simulink model "DOB_practice"  (R2021a)
settings: Solver=VariableStepAuto  StartTime=0.0  StopTime=20  RelTol=1e-3
settings Model: Creator=pyi12  LastModifiedBy=pyi12

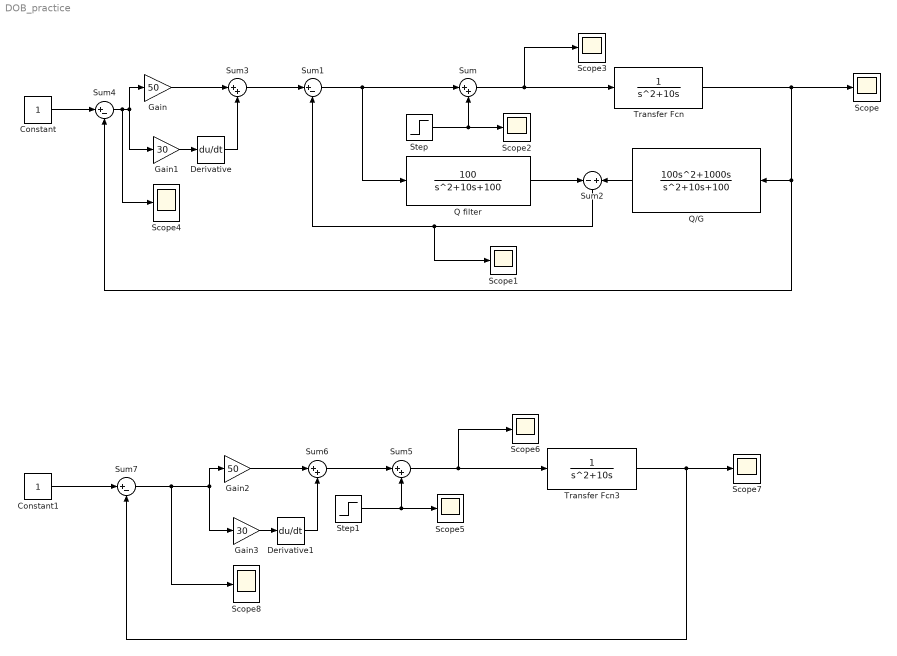
== system DOB_practice ==
  Constant : Constant
  Constant1 : Constant
  Derivative : Derivative
  Derivative1 : Derivative
  Gain : Gain  Gain=50
  Gain1 : Gain  Gain=30
  Gain2 : Gain  Gain=50
  Gain3 : Gain  Gain=30
  Q filter : TransferFcn  Numerator=[100]  Denominator=[1 10 100]
  Q/G : TransferFcn  Numerator=[100 1000 0]  Denominator=[1 10 100]
  Scope{,1..8} (9 alike) : Scope
  Step : Step  Time=0  After=5  SampleTime=0
  Step1 : Step  Time=0  After=5  SampleTime=0
  Sum{,3,5..6} (4 alike) : Sum  Inputs=|++
  Sum1 : Sum  Inputs=|+-
  Sum2 : Sum  Inputs=-+
  Sum4 : Sum  Inputs=|+-
  Sum7 : Sum  Inputs=|+-
  Transfer Fcn : TransferFcn  Denominator=[1 10 0]
  Transfer Fcn3 : TransferFcn  Denominator=[1 10 0]
  wires:
  Transfer Fcn/1 -> Sum4/2, Q/G/1, Scope/1
  Sum1/1 -> Sum/1, Q filter/1
  Q filter/1 -> Sum2/1
  Q/G/1 -> Sum2/2
  Sum2/1 -> Scope1/1, Sum1/2
  Sum/1 -> Scope3/1, Transfer Fcn/1
  Step/1 -> Scope2/1, Sum/2
  Gain/1 -> Sum3/1
  Derivative/1 -> Sum3/2
  Sum3/1 -> Sum1/1
  Sum4/1 -> Scope4/1, Gain1/1, Gain/1
  Constant/1 -> Sum4/1
  Gain1/1 -> Derivative/1
  Step1/1 -> Scope5/1, Sum5/2
  Sum5/1 -> Scope6/1, Transfer Fcn3/1
  Transfer Fcn3/1 -> Sum7/2, Scope7/1
  Gain3/1 -> Derivative1/1
  Gain2/1 -> Sum6/1
  Sum7/1 -> Scope8/1, Gain3/1, Gain2/1
  Derivative1/1 -> Sum6/2
  Sum6/1 -> Sum5/1
  Constant1/1 -> Sum7/1
